simulink library "nonTradSpoolingController_ul"  (R2018b)
settings: Solver=VariableStepAuto  StartTime=0.0  StopTime=10.0  RelTol=1e-3
undefined symbols (not defined in the file or in its folder): pathCtrl
libraries: firstOrderFilter_ul x1
settings Model: Creator=James Reed  LastModifiedBy=mcobb

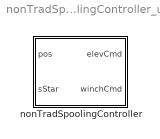
== system nonTradSpoolingController_ul ==
  nonTradSpoolingController : Subsystem

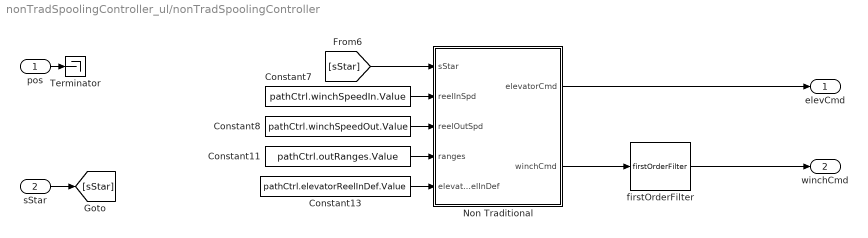
== system nonTradSpoolingController_ul/nonTradSpoolingController ==
  pos : Inport
  "sStar " : Inport  Port=2
  Constant11 : Constant  Value=pathCtrl.outRanges.Value
  Constant13 : Constant  Value=pathCtrl.elevatorReelInDef.Value
  Constant7 : Constant  Value=pathCtrl.winchSpeedIn.Value
  Constant8 : Constant  Value=pathCtrl.winchSpeedOut.Value
  Non Traditional : Stateflow chart  TreatAsAtomicUnit=on
  Terminator : Terminator
  firstOrderFilter : firstOrderFilter_ul/firstOrderFilter  tau=1  ic=0
  elevCmd : Outport
  "winchCmd " : Outport  Port=2
  wires:
  firstOrderFilter/1 -> "winchCmd "/1
  Constant13/1 -> Non Traditional/5(elevatorReelInDef)
  Constant8/1 -> Non Traditional/3(reelOutSpd)
  [sStar] -> Non Traditional/1(sStar)
  Non Traditional/1(elevatorCmd) -> elevCmd/1
  Constant11/1 -> Non Traditional/4(ranges)
  Constant7/1 -> Non Traditional/2(reelInSpd)
  Non Traditional/2(winchCmd) -> firstOrderFilter/1
  "sStar "/1 -> [sStar]
  pos/1 -> Terminator/1

== stateflow chart nonTradSpoolingController_ul/nonTradSpoolingController/Non Traditional ==
  state ReelIn
    entry:
    elevatorCmd= elevatorReelInDef;
    winchCmd = reelInSpd;
  state ReelOut
    entry:
    winchCmd = reelOutSpd;
    elevatorCmd= 0;
  (default) -> ReelOut
  ReelOut -> ReelIn : [ ~any(and(sStar>=ranges(:,1),sStar<ranges(:,2)))]
  ReelIn -> ReelOut : [any(and(sStar>=ranges(:,1),sStar<ranges(:,2)))]
  data: elevatorCmd output; sStar input; winchCmd output; reelInSpd input; reelOutSpd input; ranges input; elevatorReelInDef input
